simulink model "MOBATSim"  (R2020b)
settings: Solver=FixedStepAuto  StartTime=0.0  StopTime=Sim_t  FixedStep=0.01  MinStep=0.01  RelTol=1e-2
undefined symbols (not defined in the file): meters, Sim_Ts, Vehicle_id, Vehicles
libraries: simulink x31, robotalgslib x11, drivingvehiclecontroller x11, mpcadaslib x1, pid_lib x1
(part 5 of 5)

== system MOBATSim/Vehicle Model 8/Longitudinal and Lateral Controllers/Longitudinal Speed Control/Distance to Stop Controller1 ==
  Distance to Stop : Inport
  Compare To Constant : simulink/Logic and Bit Operations/Compare To Constant  relop=>=  const=10  OutDataTypeStr=uint8
  Gain : Gain  Gain=0.08
  Product : Product
  ref speed : Outport  VectorParamsAs1DForOutWhenUnconnected=off
  wires:
  Distance to Stop/1 -> Compare To Constant/1, Gain/1
  Gain/1 -> Product/1
  Compare To Constant/1 -> Product/2
  Product/1 -> ref speed/1

== system MOBATSim/Vehicle Model 8/Longitudinal and Lateral Controllers/Longitudinal Speed Control/Reference Acceleration Generation ==
  Driving Mode : Inport
  Speed Error : Inport  Port=2
  Actual Speed : Inport  Port=3
  Emergency Brake : Constant  Value=Vehicles(Vehicle_id).dynamics.minDeceleration
  Gear Logic : Stateflow chart  TreatAsAtomicUnit=on
  Multiport Switch3 : MultiPortSwitch  Inputs=4
  Saturation Dynamic : simulink/Discontinuities/Saturation Dynamic  OutMin=[]  OutMax=[]  OutDataTypeStr=Inherit: Same as second input  OutDataType=fixdt(1, 16)  OutScaling=2^-10  DoSatur=off
  Reference Acceleration Command : Outport  VectorParamsAs1DForOutWhenUnconnected=off
  wires:
  Driving Mode/1 -> Multiport Switch3/1
  Speed Error/1 -> Saturation Dynamic/2
  Emergency Brake/1 -> Saturation Dynamic/3, Multiport Switch3/4
  Saturation Dynamic/1 -> Multiport Switch3/5, Multiport Switch3/2, Multiport Switch3/3
  Actual Speed/1 -> Gear Logic/1(speed)
  Multiport Switch3/1 -> Reference Acceleration Command/1
  Gear Logic/1(maxAcc) -> Saturation Dynamic/1

== system MOBATSim/Vehicle Model 8/Longitudinal and Lateral Controllers/Longitudinal Speed Control/Reference speed according to the driving mode ==
  Driving Mode : Inport
  1 : Inport  Port=2
  2 : Inport  Port=3
  4 : Inport  Port=4
  Constant1 : Constant  Value=0
  Max Speed : Saturate  UpperLimit=Vehicles(Vehicle_id).dynamics.maxSpeed  LowerLimit=-100
  Multiport Switch : MultiPortSwitch  Inputs=4
  Reference Speed : Outport
  wires:
  Constant1/1 -> Multiport Switch/4
  Multiport Switch/1 -> Max Speed/1
  Driving Mode/1 -> Multiport Switch/1
  2/1 -> Multiport Switch/3
  1/1 -> Multiport Switch/2
  Max Speed/1 -> Reference Speed/1
  4/1 -> Multiport Switch/5

== system MOBATSim/Vehicle Model 9/Longitudinal and Lateral Controllers/Lateral Motion Control/Pure Pursuit ==
  pose : Inport
  speed : Inport  Port=2
  changeLane : Inport  Port=3
  MATLAB System : MATLABSystem  System=PurePursuit_WPGenerator  Vehicle_id=Vehicle_id  SimulateUsing=Interpreted execution
      mask Type: PurePursuit_WPGenerator
      mask Display:
      | image('MOBATSIM-Icon-Set_9- PurePursuit WP Generator.png');
      | port_label('input',1,'pose');
      | port_label('input',2,'speed');
      | port_label('input',3,'changeLane');
      | port_label('output',1,'nextWPs');
  Pure Pursuit : robotalgslib/Pure Pursuit  DesiredLinearVelocity=Vehicles(Vehicle_id).dynamics.maxSpeed  MaxAngularVelocity=1  LookaheadDistance=6  TargetDirPort=on  SimulateUsing=Code generation
  Terminator : Terminator
  Terminator1 : Terminator
  Wheel Steering Angle Formulation : Subsystem
  SteerCmd : Outport
  wires:
  MATLAB System/1 -> Pure Pursuit/2
  pose/1 -> Pure Pursuit/1, MATLAB System/1
  speed/1 -> MATLAB System/2
  changeLane/1 -> MATLAB System/3
  Pure Pursuit/3 -> Wheel Steering Angle Formulation/1(alpha)
  Pure Pursuit/1 -> Terminator/1
  Pure Pursuit/2 -> Terminator1/1
  Wheel Steering Angle Formulation/1(referenceYawAngle) -> SteerCmd/1

== system MOBATSim/Vehicle Model 9/Longitudinal and Lateral Controllers/Lateral Motion Control/Stanley ==
  pose : Inport
  speed : Inport  Port=2
  changeLane : Inport  Port=3
  Constant5 : Constant
  Deg to Rad : Gain  Gain=pi/180
  Lateral Controller Stanley : drivingvehiclecontroller/Lateral Controller Stanley  ModelType=Kinematic bicycle model  PositionGainF=2.5  PositionGainR=2.5  YawRateGain=0.2  DelayGain=0.2  VehicleMass=1575  Lf=1.2  Lr=1.6  TireStiffness=19000  Wheelbase=3  MaxSteeringAngle=35
      settings: SourceProductBaseCode=DR
  Stanley Reference Pose Generator : MATLABSystem  System=Stanley_RefPoseGenerator  Vehicle_id=Vehicle_id  SimulateUsing=Interpreted execution
      mask Type: Stanley_RefPoseGenerator
      mask Display:
      | image('MOBATSIM-Icon-Set_10- Stanley.png');
      | port_label('input',1,'pose');
      | port_label('input',2,'speed');
      | port_label('input',3,'changeLane');
      | port_label('output',1,'poseOut');
      | port_label('output',2,'referencePose');
  SteerCmd : Outport
  wires:
  Constant5/1 -> Lateral Controller Stanley/4
  Lateral Controller Stanley/1 -> Deg to Rad/1
  changeLane/1 -> Stanley Reference Pose Generator/3
  Stanley Reference Pose Generator/1 -> Lateral Controller Stanley/2
  Stanley Reference Pose Generator/2 -> Lateral Controller Stanley/1
  pose/1 -> Stanley Reference Pose Generator/1
  speed/1 -> Lateral Controller Stanley/3, Stanley Reference Pose Generator/2
  Deg to Rad/1 -> SteerCmd/1

== system MOBATSim/Vehicle Model 9/Longitudinal and Lateral Controllers/Longitudinal Speed Control/Distance to Stop Controller1 ==
  Distance to Stop : Inport
  Compare To Constant : simulink/Logic and Bit Operations/Compare To Constant  relop=>=  const=10  OutDataTypeStr=uint8
  Gain : Gain  Gain=0.08
  Product : Product
  ref speed : Outport  VectorParamsAs1DForOutWhenUnconnected=off
  wires:
  Distance to Stop/1 -> Compare To Constant/1, Gain/1
  Gain/1 -> Product/1
  Compare To Constant/1 -> Product/2
  Product/1 -> ref speed/1

== system MOBATSim/Vehicle Model 9/Longitudinal and Lateral Controllers/Longitudinal Speed Control/Reference Acceleration Generation ==
  Driving Mode : Inport
  Speed Error : Inport  Port=2
  Actual Speed : Inport  Port=3
  Emergency Brake : Constant  Value=Vehicles(Vehicle_id).dynamics.minDeceleration
  Gear Logic : Stateflow chart  TreatAsAtomicUnit=on
  Multiport Switch3 : MultiPortSwitch  Inputs=4
  Saturation Dynamic : simulink/Discontinuities/Saturation Dynamic  OutMin=[]  OutMax=[]  OutDataTypeStr=Inherit: Same as second input  OutDataType=fixdt(1, 16)  OutScaling=2^-10  DoSatur=off
  Reference Acceleration Command : Outport  VectorParamsAs1DForOutWhenUnconnected=off
  wires:
  Driving Mode/1 -> Multiport Switch3/1
  Speed Error/1 -> Saturation Dynamic/2
  Emergency Brake/1 -> Saturation Dynamic/3, Multiport Switch3/4
  Saturation Dynamic/1 -> Multiport Switch3/5, Multiport Switch3/2, Multiport Switch3/3
  Actual Speed/1 -> Gear Logic/1(speed)
  Multiport Switch3/1 -> Reference Acceleration Command/1
  Gear Logic/1(maxAcc) -> Saturation Dynamic/1

== system MOBATSim/Vehicle Model 9/Longitudinal and Lateral Controllers/Longitudinal Speed Control/Reference speed according to the driving mode ==
  Driving Mode : Inport
  1 : Inport  Port=2
  2 : Inport  Port=3
  4 : Inport  Port=4
  Constant1 : Constant  Value=0
  Max Speed : Saturate  UpperLimit=Vehicles(Vehicle_id).dynamics.maxSpeed  LowerLimit=-100
  Multiport Switch : MultiPortSwitch  Inputs=4
  Reference Speed : Outport
  wires:
  Constant1/1 -> Multiport Switch/4
  Multiport Switch/1 -> Max Speed/1
  Driving Mode/1 -> Multiport Switch/1
  2/1 -> Multiport Switch/3
  1/1 -> Multiport Switch/2
  Max Speed/1 -> Reference Speed/1
  4/1 -> Multiport Switch/5

== system MOBATSim/Vehicle Model 1/Longitudinal and Lateral Controllers/Lateral Motion Control/Pure Pursuit/Wheel Steering Angle Formulation ==
  note: $\delta(t)=tan^{-1} \left( \frac{2\ L\ sin(\alpha)}{l_{d}} \right)$
  alpha : Inport
  Atan : Trigonometry  Operator=atan
  Divide : Product  Inputs=*/
  Gain : Gain  Gain=2
  One over Look Ahead Distance : Constant  Value=6
  Product : Product
  Sine Wave : Sin  TimeSource=Use external signal  SampleTime=0
  Wheel Base : Constant  Value=3
  referenceYawAngle : Outport
  wires:
  Wheel Base/1 -> Gain/1
  Gain/1 -> Product/1
  alpha/1 -> Sine Wave/1
  Sine Wave/1 -> Product/2
  Product/1 -> Divide/1
  One over Look Ahead Distance/1 -> Divide/2
  Divide/1 -> Atan/1
  Atan/1 -> referenceYawAngle/1

== system MOBATSim/Vehicle Model 10/Longitudinal and Lateral Controllers/Lateral Motion Control/Pure Pursuit/Wheel Steering Angle Formulation ==
  note: $\delta(t)=tan^{-1} \left( \frac{2\ L\ sin(\alpha)}{l_{d}} \right)$
  alpha : Inport
  Atan : Trigonometry  Operator=atan
  Divide : Product  Inputs=*/
  Gain : Gain  Gain=2
  One over Look Ahead Distance : Constant  Value=6
  Product : Product
  Sine Wave : Sin  TimeSource=Use external signal  SampleTime=0
  Wheel Base : Constant  Value=3
  referenceYawAngle : Outport
  wires:
  Wheel Base/1 -> Gain/1
  Gain/1 -> Product/1
  alpha/1 -> Sine Wave/1
  Sine Wave/1 -> Product/2
  Product/1 -> Divide/1
  One over Look Ahead Distance/1 -> Divide/2
  Divide/1 -> Atan/1
  Atan/1 -> referenceYawAngle/1

== system MOBATSim/Vehicle Model 2/Longitudinal and Lateral Controllers/Lateral Motion Control/Pure Pursuit/Target direction to steering angle command ==
  note: $arctan \left( \frac{2\ L_{width}\ sin(\alpha_{dir})}{l_{d}} \right) = \delta(t)$
  alpha : Inport
  2*Wheel Base/Look ahead dist : Constant  Value=2*4/6
  Atan : Trigonometry  Operator=atan
  Product : Product
  Sin : Trigonometry
  Ref Steering Angle : Outport
  wires:
  2*Wheel Base/Look ahead dist/1 -> Product/1
  alpha/1 -> Sin/1
  Sin/1 -> Product/2
  Product/1 -> Atan/1
  Atan/1 -> Ref Steering Angle/1

== system MOBATSim/Vehicle Model 3/Longitudinal and Lateral Controllers/Lateral Motion Control/Pure Pursuit/Wheel Steering Angle Formulation ==
  note: $\delta(t)=tan^{-1} \left( \frac{2\ L\ sin(\alpha)}{l_{d}} \right)$
  alpha : Inport
  Atan : Trigonometry  Operator=atan
  Divide : Product  Inputs=*/
  Gain : Gain  Gain=2
  One over Look Ahead Distance : Constant  Value=6
  Product : Product
  Sine Wave : Sin  TimeSource=Use external signal  SampleTime=0
  Wheel Base : Constant  Value=3
  referenceYawAngle : Outport
  wires:
  Wheel Base/1 -> Gain/1
  Gain/1 -> Product/1
  alpha/1 -> Sine Wave/1
  Sine Wave/1 -> Product/2
  Product/1 -> Divide/1
  One over Look Ahead Distance/1 -> Divide/2
  Divide/1 -> Atan/1
  Atan/1 -> referenceYawAngle/1

== system MOBATSim/Vehicle Model 4/Longitudinal and Lateral Controllers/Lateral Motion Control/Pure Pursuit/Wheel Steering Angle Formulation ==
  note: $\delta(t)=tan^{-1} \left( \frac{2\ L\ sin(\alpha)}{l_{d}} \right)$
  alpha : Inport
  Atan : Trigonometry  Operator=atan
  Divide : Product  Inputs=*/
  Gain : Gain  Gain=2
  One over Look Ahead Distance : Constant  Value=6
  Product : Product
  Sine Wave : Sin  TimeSource=Use external signal  SampleTime=0
  Wheel Base : Constant  Value=3
  referenceYawAngle : Outport
  wires:
  Wheel Base/1 -> Gain/1
  Gain/1 -> Product/1
  alpha/1 -> Sine Wave/1
  Sine Wave/1 -> Product/2
  Product/1 -> Divide/1
  One over Look Ahead Distance/1 -> Divide/2
  Divide/1 -> Atan/1
  Atan/1 -> referenceYawAngle/1

== system MOBATSim/Vehicle Model 5/Longitudinal and Lateral Controllers/Lateral Motion Control/Pure Pursuit/Wheel Steering Angle Formulation ==
  note: $\delta(t)=tan^{-1} \left( \frac{2\ L\ sin(\alpha)}{l_{d}} \right)$
  alpha : Inport
  Atan : Trigonometry  Operator=atan
  Divide : Product  Inputs=*/
  Gain : Gain  Gain=2
  One over Look Ahead Distance : Constant  Value=6
  Product : Product
  Sine Wave : Sin  TimeSource=Use external signal  SampleTime=0
  Wheel Base : Constant  Value=3
  referenceYawAngle : Outport
  wires:
  Wheel Base/1 -> Gain/1
  Gain/1 -> Product/1
  alpha/1 -> Sine Wave/1
  Sine Wave/1 -> Product/2
  Product/1 -> Divide/1
  One over Look Ahead Distance/1 -> Divide/2
  Divide/1 -> Atan/1
  Atan/1 -> referenceYawAngle/1

== system MOBATSim/Vehicle Model 6/Longitudinal and Lateral Controllers/Lateral Motion Control/Pure Pursuit/Wheel Steering Angle Formulation ==
  note: $\delta(t)=tan^{-1} \left( \frac{2\ L\ sin(\alpha)}{l_{d}} \right)$
  alpha : Inport
  Atan : Trigonometry  Operator=atan
  Divide : Product  Inputs=*/
  Gain : Gain  Gain=2
  One over Look Ahead Distance : Constant  Value=6
  Product : Product
  Sine Wave : Sin  TimeSource=Use external signal  SampleTime=0
  Wheel Base : Constant  Value=3
  referenceYawAngle : Outport
  wires:
  Wheel Base/1 -> Gain/1
  Gain/1 -> Product/1
  alpha/1 -> Sine Wave/1
  Sine Wave/1 -> Product/2
  Product/1 -> Divide/1
  One over Look Ahead Distance/1 -> Divide/2
  Divide/1 -> Atan/1
  Atan/1 -> referenceYawAngle/1

== system MOBATSim/Vehicle Model 7/Longitudinal and Lateral Controllers/Lateral Motion Control/Pure Pursuit/Wheel Steering Angle Formulation ==
  note: $\delta(t)=tan^{-1} \left( \frac{2\ L\ sin(\alpha)}{l_{d}} \right)$
  alpha : Inport
  Atan : Trigonometry  Operator=atan
  Divide : Product  Inputs=*/
  Gain : Gain  Gain=2
  One over Look Ahead Distance : Constant  Value=6
  Product : Product
  Sine Wave : Sin  TimeSource=Use external signal  SampleTime=0
  Wheel Base : Constant  Value=3
  referenceYawAngle : Outport
  wires:
  Wheel Base/1 -> Gain/1
  Gain/1 -> Product/1
  alpha/1 -> Sine Wave/1
  Sine Wave/1 -> Product/2
  Product/1 -> Divide/1
  One over Look Ahead Distance/1 -> Divide/2
  Divide/1 -> Atan/1
  Atan/1 -> referenceYawAngle/1

== system MOBATSim/Vehicle Model 8/Longitudinal and Lateral Controllers/Lateral Motion Control/Pure Pursuit/Wheel Steering Angle Formulation ==
  note: $\delta(t)=tan^{-1} \left( \frac{2\ L\ sin(\alpha)}{l_{d}} \right)$
  alpha : Inport
  Atan : Trigonometry  Operator=atan
  Divide : Product  Inputs=*/
  Gain : Gain  Gain=2
  One over Look Ahead Distance : Constant  Value=6
  Product : Product
  Sine Wave : Sin  TimeSource=Use external signal  SampleTime=0
  Wheel Base : Constant  Value=3
  referenceYawAngle : Outport
  wires:
  Wheel Base/1 -> Gain/1
  Gain/1 -> Product/1
  alpha/1 -> Sine Wave/1
  Sine Wave/1 -> Product/2
  Product/1 -> Divide/1
  One over Look Ahead Distance/1 -> Divide/2
  Divide/1 -> Atan/1
  Atan/1 -> referenceYawAngle/1

== system MOBATSim/Vehicle Model 9/Longitudinal and Lateral Controllers/Lateral Motion Control/Pure Pursuit/Wheel Steering Angle Formulation ==
  note: $\delta(t)=tan^{-1} \left( \frac{2\ L\ sin(\alpha)}{l_{d}} \right)$
  alpha : Inport
  Atan : Trigonometry  Operator=atan
  Divide : Product  Inputs=*/
  Gain : Gain  Gain=2
  One over Look Ahead Distance : Constant  Value=6
  Product : Product
  Sine Wave : Sin  TimeSource=Use external signal  SampleTime=0
  Wheel Base : Constant  Value=3
  referenceYawAngle : Outport
  wires:
  Wheel Base/1 -> Gain/1
  Gain/1 -> Product/1
  alpha/1 -> Sine Wave/1
  Sine Wave/1 -> Product/2
  Product/1 -> Divide/1
  One over Look Ahead Distance/1 -> Divide/2
  Divide/1 -> Atan/1
  Atan/1 -> referenceYawAngle/1

== stateflow chart MOBATSim/Vehicle Model 6/Longitudinal and Lateral Controllers/Longitudinal Speed Control/Reference Acceleration Generation/Gear Logic ==
  settings: sampleTime=0.1
  state Gear1
    entry:
    maxAcc=6;
  state Gear2
    entry:
    maxAcc=5;
  state Gear3
    entry:
    maxAcc=3.8;
  state Gear4
    entry:
    maxAcc=3;
  state Gear5
    entry:
    maxAcc=2.2;
  state Gear6
    entry:
    maxAcc=1.4;
  (default) -> Gear1
  Gear3 -> Gear4 [order 2] : [speed>9]
  Gear4 -> Gear5 [order 1] : [speed>12]
  Gear2 -> Gear3 [order 1] : [speed>6]
  Gear5 -> Gear6 [order 2] : [speed>14]
  Gear1 -> Gear2 : [speed>3]
  Gear6 -> Gear5 : [speed<14]
  Gear4 -> Gear3 [order 2] : [speed<9]
  Gear5 -> Gear4 [order 1] : [speed<12]
  Gear2 -> Gear1 [order 2] : [speed<3]
  Gear3 -> Gear2 [order 1] : [speed<6]
  data: speed input; maxAcc output

== stateflow chart MOBATSim/Vehicle Model 7/Longitudinal and Lateral Controllers/Longitudinal Speed Control/Reference Acceleration Generation/Gear Logic ==
  settings: sampleTime=0.1
  state Gear1
    entry:
    maxAcc=6;
  state Gear2
    entry:
    maxAcc=5;
  state Gear3
    entry:
    maxAcc=3.8;
  state Gear4
    entry:
    maxAcc=3;
  state Gear5
    entry:
    maxAcc=2.2;
  state Gear6
    entry:
    maxAcc=1.4;
  (default) -> Gear1
  Gear3 -> Gear4 [order 2] : [speed>9]
  Gear4 -> Gear5 [order 1] : [speed>12]
  Gear2 -> Gear3 [order 1] : [speed>6]
  Gear5 -> Gear6 [order 2] : [speed>14]
  Gear1 -> Gear2 : [speed>3]
  Gear6 -> Gear5 : [speed<14]
  Gear4 -> Gear3 [order 2] : [speed<9]
  Gear5 -> Gear4 [order 1] : [speed<12]
  Gear2 -> Gear1 [order 2] : [speed<3]
  Gear3 -> Gear2 [order 1] : [speed<6]
  data: speed input; maxAcc output

== stateflow chart MOBATSim/Vehicle Model 8/Longitudinal and Lateral Controllers/Longitudinal Speed Control/Reference Acceleration Generation/Gear Logic ==
  settings: sampleTime=0.1
  state Gear1
    entry:
    maxAcc=6;
  state Gear2
    entry:
    maxAcc=5;
  state Gear3
    entry:
    maxAcc=3.8;
  state Gear4
    entry:
    maxAcc=3;
  state Gear5
    entry:
    maxAcc=2.2;
  state Gear6
    entry:
    maxAcc=1.4;
  (default) -> Gear1
  Gear3 -> Gear4 [order 2] : [speed>9]
  Gear4 -> Gear5 [order 1] : [speed>12]
  Gear2 -> Gear3 [order 1] : [speed>6]
  Gear5 -> Gear6 [order 2] : [speed>14]
  Gear1 -> Gear2 : [speed>3]
  Gear6 -> Gear5 : [speed<14]
  Gear4 -> Gear3 [order 2] : [speed<9]
  Gear5 -> Gear4 [order 1] : [speed<12]
  Gear2 -> Gear1 [order 2] : [speed<3]
  Gear3 -> Gear2 [order 1] : [speed<6]
  data: speed input; maxAcc output

== stateflow chart MOBATSim/Vehicle Model 9/Longitudinal and Lateral Controllers/Longitudinal Speed Control/Reference Acceleration Generation/Gear Logic ==
  settings: sampleTime=0.1
  state Gear1
    entry:
    maxAcc=6;
  state Gear2
    entry:
    maxAcc=5;
  state Gear3
    entry:
    maxAcc=3.8;
  state Gear4
    entry:
    maxAcc=3;
  state Gear5
    entry:
    maxAcc=2.2;
  state Gear6
    entry:
    maxAcc=1.4;
  (default) -> Gear1
  Gear3 -> Gear4 [order 2] : [speed>9]
  Gear4 -> Gear5 [order 1] : [speed>12]
  Gear2 -> Gear3 [order 1] : [speed>6]
  Gear5 -> Gear6 [order 2] : [speed>14]
  Gear1 -> Gear2 : [speed>3]
  Gear6 -> Gear5 : [speed<14]
  Gear4 -> Gear3 [order 2] : [speed<9]
  Gear5 -> Gear4 [order 1] : [speed<12]
  Gear2 -> Gear1 [order 2] : [speed<3]
  Gear3 -> Gear2 [order 1] : [speed<6]
  data: speed input; maxAcc output

== stateflow chart MOBATSim/Vehicle Model 10/Longitudinal and Lateral Controllers/Longitudinal Speed Control/Reference Acceleration Generation/Gear Logic ==
  settings: sampleTime=0.1
  state Gear1
    entry:
    maxAcc=6;
  state Gear2
    entry:
    maxAcc=5;
  state Gear3
    entry:
    maxAcc=3.8;
  state Gear4
    entry:
    maxAcc=3;
  state Gear5
    entry:
    maxAcc=2.2;
  state Gear6
    entry:
    maxAcc=1.4;
  (default) -> Gear1
  Gear3 -> Gear4 [order 2] : [speed>9]
  Gear4 -> Gear5 [order 1] : [speed>12]
  Gear2 -> Gear3 [order 1] : [speed>6]
  Gear5 -> Gear6 [order 2] : [speed>14]
  Gear1 -> Gear2 : [speed>3]
  Gear6 -> Gear5 : [speed<14]
  Gear4 -> Gear3 [order 2] : [speed<9]
  Gear5 -> Gear4 [order 1] : [speed<12]
  Gear2 -> Gear1 [order 2] : [speed<3]
  Gear3 -> Gear2 [order 1] : [speed<6]
  data: speed input; maxAcc output

== stateflow chart MOBATSim/Vehicle Model 1/Longitudinal and Lateral Controllers/Longitudinal Speed Control/Reference Acceleration Generation/Gear Logic ==
  settings: sampleTime=0.1
  state Gear1
    entry:
    maxAcc=6;
  state Gear2
    entry:
    maxAcc=5;
  state Gear3
    entry:
    maxAcc=3.8;
  state Gear4
    entry:
    maxAcc=3;
  state Gear5
    entry:
    maxAcc=2.2;
  state Gear6
    entry:
    maxAcc=1.4;
  (default) -> Gear1
  Gear3 -> Gear4 [order 2] : [speed>9]
  Gear4 -> Gear5 [order 1] : [speed>12]
  Gear2 -> Gear3 [order 1] : [speed>6]
  Gear5 -> Gear6 [order 2] : [speed>14]
  Gear1 -> Gear2 : [speed>3]
  Gear6 -> Gear5 : [speed<14]
  Gear4 -> Gear3 [order 2] : [speed<9]
  Gear5 -> Gear4 [order 1] : [speed<12]
  Gear2 -> Gear1 [order 2] : [speed<3]
  Gear3 -> Gear2 [order 1] : [speed<6]
  data: speed input; maxAcc output

== stateflow chart MOBATSim/Vehicle Model 2/Longitudinal and Lateral Controllers/Longitudinal Speed Control/Reference Acceleration Generation/Gear Logic ==
  settings: sampleTime=0.1
  state Gear1
    entry:
    maxAcc=6;
  state Gear2
    entry:
    maxAcc=5;
  state Gear3
    entry:
    maxAcc=3.8;
  state Gear4
    entry:
    maxAcc=3;
  state Gear5
    entry:
    maxAcc=2.2;
  state Gear6
    entry:
    maxAcc=1.4;
  (default) -> Gear1
  Gear3 -> Gear4 [order 2] : [speed>9]
  Gear4 -> Gear5 [order 1] : [speed>12]
  Gear2 -> Gear3 [order 1] : [speed>6]
  Gear5 -> Gear6 [order 2] : [speed>14]
  Gear1 -> Gear2 : [speed>3]
  Gear6 -> Gear5 : [speed<14]
  Gear4 -> Gear3 [order 2] : [speed<9]
  Gear5 -> Gear4 [order 1] : [speed<12]
  Gear2 -> Gear1 [order 2] : [speed<3]
  Gear3 -> Gear2 [order 1] : [speed<6]
  data: speed input; maxAcc output

== stateflow chart MOBATSim/Vehicle Model 3/Longitudinal and Lateral Controllers/Longitudinal Speed Control/Reference Acceleration Generation/Gear Logic ==
  settings: sampleTime=0.1
  state Gear1
    entry:
    maxAcc=6;
  state Gear2
    entry:
    maxAcc=5;
  state Gear3
    entry:
    maxAcc=3.8;
  state Gear4
    entry:
    maxAcc=3;
  state Gear5
    entry:
    maxAcc=2.2;
  state Gear6
    entry:
    maxAcc=1.4;
  (default) -> Gear1
  Gear3 -> Gear4 [order 2] : [speed>9]
  Gear4 -> Gear5 [order 1] : [speed>12]
  Gear2 -> Gear3 [order 1] : [speed>6]
  Gear5 -> Gear6 [order 2] : [speed>14]
  Gear1 -> Gear2 : [speed>3]
  Gear6 -> Gear5 : [speed<14]
  Gear4 -> Gear3 [order 2] : [speed<9]
  Gear5 -> Gear4 [order 1] : [speed<12]
  Gear2 -> Gear1 [order 2] : [speed<3]
  Gear3 -> Gear2 [order 1] : [speed<6]
  data: speed input; maxAcc output

== stateflow chart MOBATSim/Vehicle Model 4/Longitudinal and Lateral Controllers/Longitudinal Speed Control/Reference Acceleration Generation/Gear Logic ==
  settings: sampleTime=0.1
  state Gear1
    entry:
    maxAcc=6;
  state Gear2
    entry:
    maxAcc=5;
  state Gear3
    entry:
    maxAcc=3.8;
  state Gear4
    entry:
    maxAcc=3;
  state Gear5
    entry:
    maxAcc=2.2;
  state Gear6
    entry:
    maxAcc=1.4;
  (default) -> Gear1
  Gear3 -> Gear4 [order 2] : [speed>9]
  Gear4 -> Gear5 [order 1] : [speed>12]
  Gear2 -> Gear3 [order 1] : [speed>6]
  Gear5 -> Gear6 [order 2] : [speed>14]
  Gear1 -> Gear2 : [speed>3]
  Gear6 -> Gear5 : [speed<14]
  Gear4 -> Gear3 [order 2] : [speed<9]
  Gear5 -> Gear4 [order 1] : [speed<12]
  Gear2 -> Gear1 [order 2] : [speed<3]
  Gear3 -> Gear2 [order 1] : [speed<6]
  data: speed input; maxAcc output

== stateflow chart MOBATSim/Vehicle Model 5/Longitudinal and Lateral Controllers/Longitudinal Speed Control/Reference Acceleration Generation/Gear Logic ==
  settings: sampleTime=0.1
  state Gear1
    entry:
    maxAcc=6;
  state Gear2
    entry:
    maxAcc=5;
  state Gear3
    entry:
    maxAcc=3.8;
  state Gear4
    entry:
    maxAcc=3;
  state Gear5
    entry:
    maxAcc=2.2;
  state Gear6
    entry:
    maxAcc=1.4;
  (default) -> Gear1
  Gear3 -> Gear4 [order 2] : [speed>9]
  Gear4 -> Gear5 [order 1] : [speed>12]
  Gear2 -> Gear3 [order 1] : [speed>6]
  Gear5 -> Gear6 [order 2] : [speed>14]
  Gear1 -> Gear2 : [speed>3]
  Gear6 -> Gear5 : [speed<14]
  Gear4 -> Gear3 [order 2] : [speed<9]
  Gear5 -> Gear4 [order 1] : [speed<12]
  Gear2 -> Gear1 [order 2] : [speed<3]
  Gear3 -> Gear2 [order 1] : [speed<6]
  data: speed input; maxAcc output
